simulink model "cesna_a_37"  (Simulink 7.6)
settings: Solver=ode45  StartTime=0.0  StopTime=200  RelTol=1e-3
model workspace (MAT data in the model file):
  CD_p : Simulink.Parameter (value not decoded)
  CL_p : Simulink.Parameter (value not decoded)
  CY_p : Simulink.Parameter (value not decoded)
  Clm_p : Simulink.Parameter (value not decoded)
  Cmm_p : Simulink.Parameter (value not decoded)
  Cnm_p : Simulink.Parameter (value not decoded)
  S : Simulink.Parameter (value not decoded)
  cbar : Simulink.Parameter (value not decoded)
  b : Simulink.Parameter (value not decoded)
  m : Simulink.Parameter (value not decoded)
  ho : Simulink.Parameter (value not decoded)
  Vo : Simulink.Parameter (value not decoded)
  Ts : Simulink.Parameter (value not decoded)
undefined symbols (not defined in the file): A, alpha_trim, B, C, D, F_T_trim
libraries: simulink x3, Airframes x1
(part 1 of 2)
settings Model: Creator=Administrator  LastModifiedBy=jporter
settings DebuggingCC: StrictBusMsg=Warning
settings SFSimCC: SimParseCustomCode=off

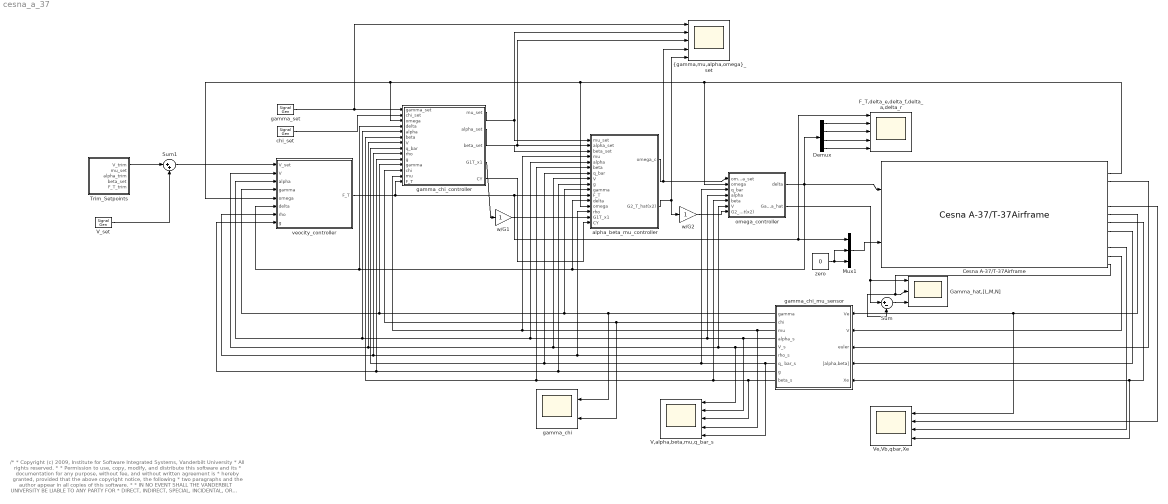
== system cesna_a_37 ==
  note: /*
      |  * Copyright (c) 2009, Institute for Software Integrated Systems, Vanderbilt University
      |  * All rights reserved.
      |  *
      |  * Permission to use, copy, modify, and distribute this software and its
      |  * documentation for any purpose, without fee, and without written agreement is
      |  * hereby granted, provided that the above copyright notice, the following
      |  * two paragraphs and the author appear in all copies of this software.
      |  *
      |  * IN NO EVENT SHALL THE VANDERBILT UNIVERSITY BE LIABLE TO ANY PARTY FOR
      |  * DIRECT, INDIRECT, SPECIAL, INCIDENTAL, OR CONSEQUENTIAL DAMAGES ARISING OUT
      |  * OF THE USE OF THIS SOFTWARE AND ITS DOCUMENTATION, EVEN IF THE VANDERBILT
      |  * UNIVERSITY HAS BEEN ADVISED OF THE POSSIBILITY OF SUCH DAMAGE.
      |  *
      |  * THE VANDERBILT UNIVERSITY SPECIFICALLY DISCLAIMS ANY WARRANTIES,
      |  * INCLUDING, BUT NOT LIMITED TO, THE IMPLIED WARRANTIES OF MERCHANTABILITY
      |  * AND FITNESS FOR A PARTICULAR PURPOSE.  THE SOFTWARE PROVIDED HEREUNDER IS
      |  * ON AN "AS IS" BASIS, AND THE VANDERBILT UNIVERSITY HAS NO OBLIGATION TO
      |  * PROVIDE MAINTENANCE, SUPPORT, UPDATES, ENHANCEMENTS, OR MODIFICATIONS.
      |  *
      |  * @author Nicholas Kottenstette
      |  * NB: Some of the atmospheric models (not including wind disturbance models) and drag-forc models including the
      | *  general aircraft interface description are for a large part a result of Giampiero Campa work with airlib, however,
      | *  equations of motion are determined using the standard 6-dof dynamic model after determening the respective
      | *  body forces applied to the aircraft not via the aerodynamic equations of motion involving angle of attack, slide-slip
      | * angle, etc.  Wind shear models and discrete-time gust models are based on the MIL–F–8785C specification.
      |  */
  Cesna A-37/T-37Airframe : Airframes/Cesna A-37//T-37Airframe  SystemSampleTime=-1  trim_enable=off  XYZe_0=[0,0,-1000]  V=Vo  Vb_0=Vo*[1,0,.0184]  euler_0=[0,.018,0]  omega_0=zeros(3,1)  M=.4535959237*6360  I=1.35581795*[7.99e3,0,2.34e2;0,3.33e3,0;2.34e2,0,1.12e4]  b=.3048*33.8  cbar=.3048*5.47  S=(.3048^2)*182  CG=[0,0,0]  CP=[0,0,0]  CD_p="[0.048,  0.384,  0,  0,  0]"  CL_p="[0.2,   5.15,    4.1,   0.5,   0]"  CY_p="[0,  -0.346,  -0.0827,  0.3,  0.0,  0.2]"  Clm_p="[0, -0.0944,  -0.442,  0.0926,  -0.181,  0.015]"  Cmm_p="[0.025, -0.7,  -14.9,  -1.12,  0]"  Cnm_p="[0,  0.1106, -0.0243,  -0.139,  0.0254,  -0.0365]"  delta_f=0  k_wind=on
  Demux : Demux
  F_T,delta_e,delta_f,delta_a,delta_r : Scope  NumInputPorts=5
      settings: YMin=0~-1.73472e-018~-1~-0.3~-0.175  YMax=17500~0.04~1~0.05~0.025  SaveName=actuator_s  SampleInput=on  SampleTime=0.05
  Gamma_hat,[L,M,N] : Scope  NumInputPorts=3
      settings: YMin=-1.5~-1.5~-3e-007  YMax=4~4~1.5e-007  SaveName=ScopeData12  SampleInput=on  SampleTime=0.01
  Mux1 : Mux  Inputs=3
  Sum : Sum  Inputs=|+-
  Sum1 : Sum  Inputs=|++
  Trim_Setpoints : Subsystem  mask{CD_p=CD_p, CL_p=CL_p, Cmm_p=Cmm_p, S=S, V=Vo, h=ho, m=m, delta_f=0}
      mask prompts: CD_p "Drag Parameters:CD_p=[CDo,CDa,CDq,CDde,CDin]"; CL_p "Lift Parameters:CL_p=[CLo,CLa,CLq,CLde,CLin]"; Cmm_p "m-moment (about-y_b) Parameters:Cmm_p=[Cmo,Cma,Cmq,Cmde,Cmin]"; S "Wing Area [S] (meters^2)"; V "Trim Velocity [V] (meters/s)"; h "Altitude [h] (meters)"; m "Mass [m] (kg)"; delta_f "delta_f [delta_f] (rad)"
      mask init:
      | [F_T_trim,alpha_trim,delta_e_trim,Sol] = fixed_wing_trim(CD_p,CL_p,Cmm_p,S,V,h,m,delta_f,[],false);
  V,alpha,beta,mu,q_bar_s : Scope  NumInputPorts=5
      settings: YMin=110~-0.05~-0.03~-0.5~6000  YMax=160~0.03~0.015~0.7~13000  SampleInput=on  SampleTime=0.04
  V_set : SignalGenerator  Amplitude=30  Frequency=.01
  Ve,Vb,qbar,Xe : Scope  NumInputPorts=4
      settings: YMin=-25~-25~12000~-1500  YMax=175~200~19000~4000  SaveName=ScopeData2  SampleInput=on  SampleTime=0.05
  alpha_beta_mu_controller : Subsystem  mask{CD_p=CD_p, CL_p=CL_p, CY_p=CY_p, S=S, b=b, cbar=cbar, m=m, K_2=[1,1,1]*1, Ts=Ts}
      mask prompts: CD_p "Drag Parameters:CD_p=[CDo,CDa,CDq,CDde,CDin]"; CL_p "Lift Parameters:CL_p=[CLo,CLa,CLq,CLde,CLin]"; CY_p "Y-Drag Parameters:CY_p=[CYo,CYb,CYp,CYr,CYda,CYdr]"; S "Wing Area [S] (meters^2)"; b "Wing Span [b] (meters)"; cbar "MAC [cbar] (meters)"; m "mass [m] (kg)"; Ts "Sample Time [Ts] (seconds)"
      mask init:
      | CDo=CD_p(1);
      | CDa=CD_p(2);
      | CDq=CD_p(3);
      | CDde=CD_p(4);
      | CDin=CD_p(5);
      | CLo=CL_p(1);
      | CLa=CL_p(2);
      | CLq=CL_p(3);
      | CLde=CL_p(4);
      | CLin=CL_p(5);
      | CYo=CY_p(1);
      | CYb=CY_p(2);
      | CYp=CY_p(3);
      | CYr=CY_p(4);
      | CYda=CY_p(5);
      | CYdr=CY_p(6);
  chi_set : SignalGenerator  Amplitude=.5  Frequency=.01
  gamma_chi : Scope  NumInputPorts=2
      settings: YMin=-0.1~-0.35  YMax=0.125~0.55  SaveName=ScopeData5  SampleInput=on  SampleTime=0.05
  gamma_chi_controller : Subsystem  mask{CL_p=CL_p, CY_p=CY_p, S=S, b=b, cbar=cbar, m=m, k_g=1, k_chi=.5, Ts=Ts}
      mask prompts: CL_p "Lift Parameters:CL_p=[CLo,CLa,CLq,CLde,CLin]"; CY_p "Y-Drag Parameters:CY_p=[CYo,CYb,CYp,CYr,CYda,CYdr]"; S "Wing Area [S] (meters^2)"; b "Wing Span [b] (meters)"; cbar "MAC [cbar] (meters)"; m "mass [m] (kg)"; Ts "Sample Period (s) [Ts]"
      mask init:
      | %CDo=CD_p(1);
      | %CDa=CD_p(2);
      | %CDq=CD_p(3);
      | %CDde=CD_p(4);
      | %CDin=CD_p(5);
      | CLo=CL_p(1);
      | CLa=CL_p(2);
      | CLq=CL_p(3);
      | CLde=CL_p(4);
      | CLin=CL_p(5);
      | CYo=CY_p(1);
      | CYb=CY_p(2);
      | CYp=CY_p(3);
      | CYr=CY_p(4);
      | CYda=CY_p(5);
      | CYdr=CY_p(6);
  gamma_chi_mu_sensor : Subsystem  mask{Ts=Ts}
      mask prompts: Ts "Sample Period (s) [Ts]"
  gamma_set : SignalGenerator  Amplitude=.1  Frequency=1/40
  omega_controller : Subsystem  mask{S=S, cbar=cbar, b=b, Clm_p=Clm_p, Cmm_p=Cmm_p, Cnm_p=Cnm_p, q_bar_nom=.5*1.225*Vo^2, k_o=[1,1,1]*1, Ts=Ts, I=1.35581795*[7.99e3,0,2.34e2;0,3.33e3,0;2.34e2,0,1.12e4]}
      mask prompts: S "Wing Area [S] (meters^2)"; cbar "MAC [cbar] (meters)"; b "Wing Span [b] (meters)"; Clm_p "l-moment (about x_b) Parameters: Clm_p=[Clo,Clb,Clp,Clr,Clda,Cldr]"; Cmm_p "m-moment (about-y_b) Parameters: Cmm_p=[Cmo,Cma,Cmq,Cmde,Cmin]"; Cnm_p "n-moment (about-z_b) Parameters:Cnm_p=[Cno,Cnb,Cnp,Cnr,Cnda,Cndr]"; Ts "Sample Period [Ts] (seconds)"; I "Inertial Matrix I"
      mask init:
      | Clo=Clm_p(1);
      | Clb=Clm_p(2);
      | Clp=Clm_p(3);
      | Clr=Clm_p(4);
      | Clda=Clm_p(5);
      | Cldr=Clm_p(6);
      | Cno=Cnm_p(1);
      | Cnb=Cnm_p(2);
      | Cnp=Cnm_p(3);
      | Cnr=Cnm_p(4);
      | Cnda=Cnm_p(5);
      | Cndr=Cnm_p(6);
      | Cmo=Cmm_p(1);
      | Cma=Cmm_p(2);
      | Cmq=Cmm_p(3);
      | Cmde=Cmm_p(4);
      | Cmin=Cmm_p(5);
  veocity_controller : Subsystem  mask{Ts=Ts, K_I=2, omega_d=1, CD_p=CD_p, CL_p=CL_p, Cmm_p=Cmm_p, S=S, V=Vo, h=ho, m=m, delta_f=0, cbar=cbar}
      mask prompts: Ts "Sample Period (s) [Ts]"; omega_d "omega_d (rad/s)"; CD_p "Drag Parameters:CD_p=[CDo,CDa,CDq,CDde,CDin]"; CL_p "Lift Parameters:CL_p=[CLo,CLa,CLq,CLde,CLin]"; Cmm_p "m-moment (about-y_b) Parameters:Cmm_p=[Cmo,Cma,Cmq,Cmde,Cmin]"; S "Wing Area (m^2): [S]"; V "Initial Trim Velocity [V] (meters/s)"; h "Initial Altitude [h] (meters)"; m "mass: (kg) [m]"; delta_f "delta_f [delta_f] (rad)"; cbar "MAC (m): [cbar]"
      mask init:
      | CDo=CD_p(1);
      | CDa=CD_p(2);
      | CDq=CD_p(3);
      | CDde=CD_p(4);
      | CDin=CD_p(5);
      | omega_n=pi/Ts;
      | [F_T_trim,alpha_trim,delta_e_trim,Sol] = fixed_wing_trim(CD_p,CL_p,Cmm_p,S,V,h,m,delta_f,[],false);
      | %Determine gravity and density at h
      | Po = 101325; %standard pressure [Pa]
      | To = 288.15; %standard temperature [Kelvin]
      | L = 6.5; %Kelvin/km
      | M = 28.9644; %gm/mol
      | R = 8.31432; %J/(mol-Kelvin)
      | g = 9.80665*((6356e3/(6356e3+h))^2);
      | T = To - 1.0e-3*L*h;
      | ps = Po*(T/To)^((g*M)/(R*L));   %Pressure at h
      | rho = ps/((1000*R/M)*T);
      | %Determine controller offset force
      | q_bar=.5*rho*V^2;
      | dF_T=-V*m*omega_d+q_bar*S*(CDa*alpha_trim+CDde*delta_e_trim+CDin*delta_f+CDo);
      | F_TI=F_T_trim-dF_T;
  w/G1 : Gain
  w/G2 : Gain
  zero : Constant  Value=0  SampleTime=Ts
  "{gamma,mu,alpha,omega}_set" : Scope  NumInputPorts=5
      settings: YMin=-0.1~-0.5~-0.03~-0.3~-0.3  YMax=0.1~0.9~0.03~0.3~0.3  SaveName=ScopeData4  SampleInput=on  SampleTime=0.05
  wires:
  gamma_chi_mu_sensor/1(gamma) -> veocity_controller/4(gamma), gamma_chi_controller/11(gamma), alpha_beta_mu_controller/10(gamma), gamma_chi/1
  Cesna A-37/T-37Airframe/7 -> gamma_chi_mu_sensor/1(Ve), Ve,Vb,qbar,Xe/1
  Cesna A-37/T-37Airframe/12 -> gamma_chi_mu_sensor/2(V)
  Cesna A-37/T-37Airframe/3 -> gamma_chi_mu_sensor/3(euler)
  Cesna A-37/T-37Airframe/9 -> gamma_chi_mu_sensor/4("[alpha,beta]")
  gamma_chi_mu_sensor/5(V_s) -> V,alpha,beta,mu,q_bar_s/1, alpha_beta_mu_controller/8(V), veocity_controller/2(V), gamma_chi_controller/7(V), omega_controller/6(V)
  gamma_chi_mu_sensor/4(alpha_s) -> omega_controller/4(alpha), alpha_beta_mu_controller/5(alpha), veocity_controller/3(alpha), gamma_chi_controller/5(alpha), V,alpha,beta,mu,q_bar_s/2
  Cesna A-37/T-37Airframe/8 -> gamma_chi_mu_sensor/5(Xe), Ve,Vb,qbar,Xe/4
  Cesna A-37/T-37Airframe/2 -> omega_controller/2(omega), alpha_beta_mu_controller/13(omega), veocity_controller/5(omega), gamma_chi_controller/3(omega)
  gamma_chi_mu_sensor/6(rho_s) -> alpha_beta_mu_controller/14(rho), veocity_controller/7(rho), gamma_chi_controller/9(rho)
  gamma_chi_mu_sensor/8(g) -> alpha_beta_mu_controller/9(g), veocity_controller/8(g), gamma_chi_controller/10(g)
  veocity_controller/1(F_T) -> alpha_beta_mu_controller/11(F_T), Mux1/1, F_T,delta_e,delta_f,delta_a,delta_r/1, gamma_chi_controller/14(F_T)
  omega_controller/1(delta) -> Cesna A-37/T-37Airframe/1, Demux/1, alpha_beta_mu_controller/12(delta), veocity_controller/6(delta), gamma_chi_controller/4(delta)
  gamma_chi_mu_sensor/7(q_ bar_s) -> V,alpha,beta,mu,q_bar_s/5, omega_controller/3(q_bar), alpha_beta_mu_controller/7(q_bar), gamma_chi_controller/8(q_bar)
  gamma_chi_mu_sensor/9(beta_s) -> omega_controller/5(beta), alpha_beta_mu_controller/6(beta), gamma_chi_controller/6(beta), V,alpha,beta,mu,q_bar_s/3
  alpha_beta_mu_controller/1(omega_c) -> omega_controller/1(omega_set), "{gamma,mu,alpha,omega}_set"/4
  gamma_chi_mu_sensor/3(mu) -> V,alpha,beta,mu,q_bar_s/4, alpha_beta_mu_controller/4(mu), gamma_chi_controller/13(mu)
  Demux/1 -> F_T,delta_e,delta_f,delta_a,delta_r/2
  Demux/2 -> F_T,delta_e,delta_f,delta_a,delta_r/3
  Demux/3 -> F_T,delta_e,delta_f,delta_a,delta_r/4
  Demux/4 -> F_T,delta_e,delta_f,delta_a,delta_r/5
  Cesna A-37/T-37Airframe/6 -> Ve,Vb,qbar,Xe/2
  Cesna A-37/T-37Airframe/11 -> Ve,Vb,qbar,Xe/3
  Mux1/1 -> Cesna A-37/T-37Airframe/2
  zero/1 -> Mux1/3, Mux1/2
  gamma_chi_mu_sensor/2(chi) -> gamma_chi/2, gamma_chi_controller/12(chi)
  gamma_chi_controller/2(alpha_set) -> alpha_beta_mu_controller/2(alpha_set), "{gamma,mu,alpha,omega}_set"/3
  gamma_chi_controller/1(mu_set) -> alpha_beta_mu_controller/1(mu_set), "{gamma,mu,alpha,omega}_set"/2
  gamma_chi_controller/3(beta_set) -> alpha_beta_mu_controller/3(beta_set)
  gamma_set/1 -> gamma_chi_controller/1(gamma_set), "{gamma,mu,alpha,omega}_set"/1
  chi_set/1 -> gamma_chi_controller/2(chi_set)
  Cesna A-37/T-37Airframe/13 -> Gamma_hat,[L,M,N]/2, Sum/2
  omega_controller/2(Gamma_hat) -> Gamma_hat,[L,M,N]/1, Sum/1
  Sum/1 -> Gamma_hat,[L,M,N]/3
  Trim_Setpoints/1(V_trim) -> Sum1/1
  Sum1/1 -> veocity_controller/1(V_set)
  V_set/1 -> Sum1/2
  gamma_chi_controller/4(G1T_x1) -> w/G1/1
  alpha_beta_mu_controller/2(G2_T_hat(x2)) -> "{gamma,mu,alpha,omega}_set"/5, w/G2/1
  w/G2/1 -> omega_controller/7(G2_T_hat(x2))
  w/G1/1 -> alpha_beta_mu_controller/15(G1T_x1)
  gamma_chi_controller/5(CY) -> alpha_beta_mu_controller/16(CY)

== system cesna_a_37/Trim_Setpoints ==
  Constant : Constant  Value=0
  V_trim_c : Constant  Value=V
  alpha_trim_c : Constant  Value=alpha_trim
  alpha_trim_c1 : Constant  Value=F_T_trim
  V_trim : Outport
  mu_set : Outport  Port=2
  alpha_trim : Outport  Port=3
  beta_set : Outport  Port=4
  F_T_trim : Outport  Port=5
  wires:
  Constant/1 -> mu_set/1, beta_set/1
  V_trim_c/1 -> V_trim/1
  alpha_trim_c/1 -> alpha_trim/1
  alpha_trim_c1/1 -> F_T_trim/1

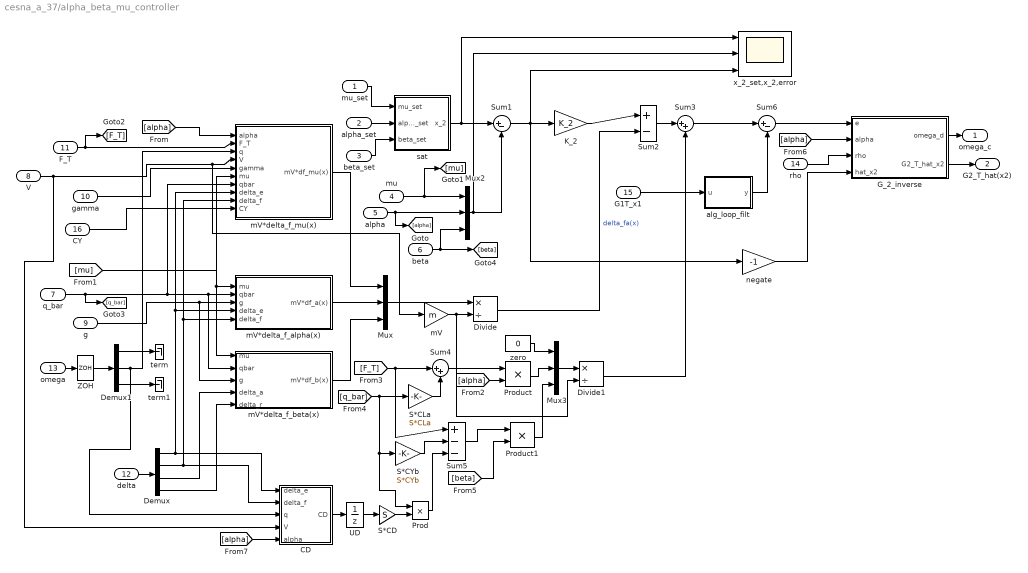
== system cesna_a_37/alpha_beta_mu_controller ==
  mu_set : Inport
  alpha_set : Inport  Port=2
  beta_set : Inport  Port=3
  mu : Inport  Port=4
  alpha : Inport  Port=5
  beta : Inport  Port=6
  q_bar : Inport  Port=7
  V : Inport  Port=8
  g : Inport  Port=9
  gamma : Inport  Port=10
  F_T : Inport  Port=11
  delta : Inport  Port=12
  omega : Inport  Port=13
  rho : Inport  Port=14
  G1T_x1 : Inport  Port=15
  CY : Inport  Port=16
  CD : Subsystem
  Demux : Demux
  Demux1 : Demux  Outputs=3
  Divide : Product  Inputs=*/
  Divide1 : Product  Inputs=*/
  G_2_inverse : Stateflow chart  TreatAsAtomicUnit=on
  K_2 : Gain  Gain=K_2
  Mux : Mux  Inputs=3
  Mux2 : Mux  Inputs=3
  Mux3 : Mux  Inputs=3
  Prod : Product  RndMeth=Zero
  Product : Product  RndMeth=Zero
  Product1 : Product  RndMeth=Zero
  S*CD : Gain  Gain=S
  S*CLa : Gain  Gain=S*CLa
  S*CYb : Gain  Gain=S*CYb
  Sum1 : Sum  Inputs=|+-
  Sum2 : Sum  Inputs=|+-
  Sum3 : Sum  Inputs=|++
  Sum4 : Sum  Inputs=|++
  Sum5 : Sum  Inputs=|+--
  Sum6 : Sum  Inputs=|+-
  UD : UnitDelay  SampleTime=-1
  ZOH : ZeroOrderHold  SampleTime=Ts
  alg_loop_filt : Subsystem
  mV : Gain  Gain=m
  mV*delta_f_alpha(x) : Subsystem
  mV*delta_f_beta(x) : Subsystem
  mV*delta_f_mu(x) : Subsystem
  negate : Gain  Gain=-1
  sat : Subsystem
  term : Terminator
  term1 : Terminator
  x_2_set,x_2,error : Scope  NumInputPorts=3
      settings: YMin=-0.4~-0.4~-0.15  YMax=0.6~0.5~0.45  SaveName=x2_s  SampleInput=on  SampleTime=0.05
  zero : Constant  Value=0
  omega_c : Outport
  G2_T_hat(x2) : Outport  Port=2
  wires:
  g/1 -> mV*delta_f_alpha(x)/3(g), mV*delta_f_beta(x)/3(g)
  q_bar/1 -> mV*delta_f_alpha(x)/2(qbar), mV*delta_f_beta(x)/2(qbar), mV*delta_f_mu(x)/7(qbar), [q_bar]
  delta/1 -> Demux/1
  Demux/1 -> mV*delta_f_alpha(x)/4(delta_e), mV*delta_f_mu(x)/8(delta_e), CD/1(delta_e)
  Demux/2 -> mV*delta_f_alpha(x)/5(delta_f), mV*delta_f_mu(x)/9(delta_f), CD/2(delta_f)
  Demux/3 -> mV*delta_f_beta(x)/4(delta_a)
  Demux/4 -> mV*delta_f_beta(x)/5(delta_r)
  V/1 -> mV*delta_f_mu(x)/4(V), mV/1, CD/4(V)
  F_T/1 -> mV*delta_f_mu(x)/2(F_T), [F_T]
  gamma/1 -> mV*delta_f_mu(x)/5(gamma)
  omega/1 -> ZOH/1
  Demux1/2 -> mV*delta_f_mu(x)/3(q), CD/3(q)
  mV*delta_f_alpha(x)/1(mV*df_a(x)) -> Mux/2
  mV*delta_f_mu(x)/1(mV*df_mu(x)) -> Mux/1
  mV*delta_f_beta(x)/1(mV*df_b(x)) -> Mux/3
  Mux/1 -> Divide/1
  mV/1 -> Divide/2, Divide1/2
  alpha/1 -> [alpha], Mux2/2
  beta/1 -> [beta], Mux2/3
  mu/1 -> [mu], Mux2/1
  Mux2/1 -> x_2_set,x_2,error/2, Sum1/2
  Sum1/1 -> K_2/1, negate/1, x_2_set,x_2,error/3
  G_2_inverse/1(omega_d) -> omega_c/1
  rho/1 -> G_2_inverse/3(rho)
  ZOH/1 -> Demux1/1
  Demux1/3 -> term1/1
  Demux1/1 -> term/1
  [alpha] -> mV*delta_f_mu(x)/1(alpha)
  [mu] -> mV*delta_f_mu(x)/6(mu), mV*delta_f_beta(x)/1(mu), mV*delta_f_alpha(x)/1(mu)
  Sum2/1 -> Sum3/1
  zero/1 -> Mux3/1
  Mux3/1 -> Divide1/1
  Divide1/1 -> Sum3/2
  [q_bar] -> S*CLa/1, S*CYb/1, Prod/1
  [F_T] -> Sum5/1, Sum4/1
  S*CLa/1 -> Sum4/2
  Sum4/1 -> Product/1
  Product/1 -> Mux3/2
  [alpha] -> Product/2
  S*CYb/1 -> Sum5/2
  [beta] -> Product1/2
  Product1/1 -> Mux3/3
  Sum5/1 -> Product1/1
  [alpha] -> G_2_inverse/2(alpha)
  mu_set/1 -> sat/1(mu_set)
  alpha_set/1 -> sat/2(alpha_set)
  beta_set/1 -> sat/3(beta_set)
  Sum3/1 -> Sum6/1
  Sum6/1 -> G_2_inverse/1(e)
  G_2_inverse/2(G2_T_hat_x2) -> G2_T_hat(x2)/1
  negate/1 -> G_2_inverse/4(hat_x2)
  CY/1 -> mV*delta_f_mu(x)/10(CY)
  alg_loop_filt/1(y) -> Sum6/2
  G1T_x1/1 -> alg_loop_filt/1(u)
  CD/1(CD) -> UD/1
  [alpha] -> CD/5(alpha)
  K_2/1 -> Sum2/1
  Divide/1 -> Sum2/2  "delta_fa(x)"
  sat/1(x_2) -> Sum1/1, x_2_set,x_2,error/1
  S*CD/1 -> Prod/2
  Prod/1 -> Sum5/3
  UD/1 -> S*CD/1

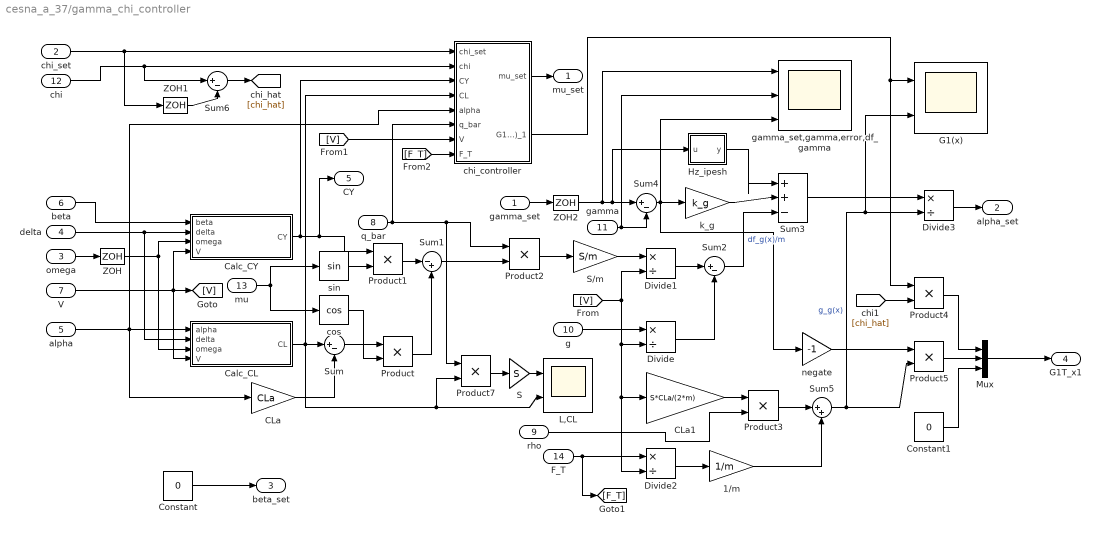
== system cesna_a_37/gamma_chi_controller ==
  gamma_set : Inport
  chi_set : Inport  Port=2
  omega : Inport  Port=3
  delta : Inport  Port=4
  alpha : Inport  Port=5
  beta : Inport  Port=6
  V : Inport  Port=7
  q_bar : Inport  Port=8
  rho : Inport  Port=9
  g : Inport  Port=10
  gamma : Inport  Port=11
  chi : Inport  Port=12
  mu : Inport  Port=13
  F_T : Inport  Port=14
  1/m : Gain  Gain=1/m
  CLa : Gain  Gain=CLa
  CLa1 : Gain  Gain=S*CLa/(2*m)
  Calc_CL : Subsystem
  Calc_CY : Subsystem
  Constant : Constant  Value=0
  Constant1 : Constant  Value=0
  Divide{,1..3} (4 alike) : Product  Inputs=*/
  G1(x) : Scope  NumInputPorts=2
      settings: YMin=0.055~1.65  YMax=0.13~2.4  SaveName=ScopeData10  SampleInput=on  SampleTime=0.05
  Hz_ipesh : Subsystem  mask{num=[1,0], den=[10*Ts/pi,1], Ts=Ts, y0=0}
      mask prompts: num "Hs num [num]"; den "Hs den [den]"; Ts "Sample Period (s) [Ts]"; y0 "y0 (N)"
      mask init:
      | Hs=tf(num,den);
      | Hz=ipesh_transform(Hs,Ts);
      | [A,B,C,D]=tf2ss(Hz.num{1},Hz.den{1});
      | x0=y0/C;
  L,CL : Scope  NumInputPorts=2
      settings: YMin=-5000~-0.025  YMax=70000~0.35  SaveName=ScopeData14  SampleInput=on  SampleTime=0.05
  Mux : Mux  Inputs=3
  Product{,1..5,7} (7 alike) : Product  RndMeth=Zero
  S : Gain  Gain=S
  S/m : Gain  Gain=S/m
  Sum{,2,4,6} (4 alike) : Sum  Inputs=|+-
  Sum1 : Sum  Inputs=|-+
  Sum3 : Sum  Inputs=|++-
  Sum5 : Sum  Inputs=|++
  ZOH : ZeroOrderHold  SampleTime=Ts
  ZOH1 : ZeroOrderHold  SampleTime=Ts
  ZOH2 : ZeroOrderHold  SampleTime=Ts
  chi_controller : Subsystem
  cos : Trigonometry  Operator=cos
  gamma_set,gamma,error,df_gamma : Scope  NumInputPorts=3
      settings: YMin=-0.1~-0.125~-0.015  YMax=0.1~0.125~0.04  SaveName=gamma_s  SampleInput=on  SampleTime=0.05
  k_g : Gain  Gain=k_g
  negate : Gain  Gain=-1
  sin : Trigonometry
  mu_set : Outport
  alpha_set : Outport  Port=2
  beta_set : Outport  Port=3
  G1T_x1 : Outport  Port=4
  CY : Outport  Port=5
  wires:
  alpha/1 -> Calc_CL/1(alpha), CLa/1, chi_controller/5(alpha)
  delta/1 -> Calc_CY/2(delta), Calc_CL/2(delta)
  beta/1 -> Calc_CY/1(beta)
  omega/1 -> ZOH/1
  V/1 -> Calc_CL/4(V), Calc_CY/4(V), [V]
  Calc_CL/1(CL) -> chi_controller/4(CL), Sum/1, L,CL/2, Product7/2
  CLa/1 -> Sum/2
  g/1 -> Divide/1
  Sum/1 -> Product/1
  mu/1 -> sin/1, cos/1
  cos/1 -> Product/2
  sin/1 -> Product1/2
  Calc_CY/1(CY) -> chi_controller/3(CY), Product1/1, CY/1
  Product1/1 -> Sum1/1
  Product/1 -> Sum1/2
  Sum1/1 -> Product2/2
  q_bar/1 -> chi_controller/6(q_bar), Product2/1, Product7/1
  Product2/1 -> S/m/1
  S/m/1 -> Divide1/1
  [V] -> Divide1/2, Divide/2, CLa1/1, Divide2/2
  Divide1/1 -> Sum2/1
  Divide/1 -> Sum2/2
  gamma_set/1 -> ZOH2/1
  gamma/1 -> gamma_set,gamma,error,df_gamma/2, Sum4/2
  Sum4/1 -> k_g/1, gamma_set,gamma,error,df_gamma/3, negate/1
  F_T/1 -> Divide2/1, [F_T]
  Divide2/1 -> 1/m/1
  1/m/1 -> Sum5/2
  CLa1/1 -> Product3/1
  rho/1 -> Product3/2
  Product3/1 -> Sum5/1
  Sum3/1 -> Divide3/1
  Sum5/1 -> Divide3/2, G1(x)/2, Product5/2  "g_g(x)"
  Divide3/1 -> alpha_set/1
  chi_set/1 -> chi_controller/1(chi_set), ZOH1/1
  chi/1 -> chi_controller/2(chi), Sum6/1
  Constant/1 -> beta_set/1
  ZOH/1 -> Calc_CY/3(omega), Calc_CL/3(omega)
  ZOH2/1 -> gamma_set,gamma,error,df_gamma/1, Sum4/1, Hz_ipesh/1(u)
  [V] -> chi_controller/7(V)
  [F_T] -> chi_controller/8(F_T)
  chi_controller/1(mu_set) -> mu_set/1
  Sum2/1 -> Sum3/3  "df_g(x)/m"
  k_g/1 -> Sum3/2
  Hz_ipesh/1(y) -> Sum3/1
  chi_controller/2(G1(x)_1) -> G1(x)/1, Product4/1
  [chi_hat] -> Product4/2
  negate/1 -> Product5/1
  Mux/1 -> G1T_x1/1
  Product4/1 -> Mux/1
  Product5/1 -> Mux/2
  Constant1/1 -> Mux/3
  Sum6/1 -> [chi_hat]
  ZOH1/1 -> Sum6/2
  Product7/1 -> S/1
  S/1 -> L,CL/1

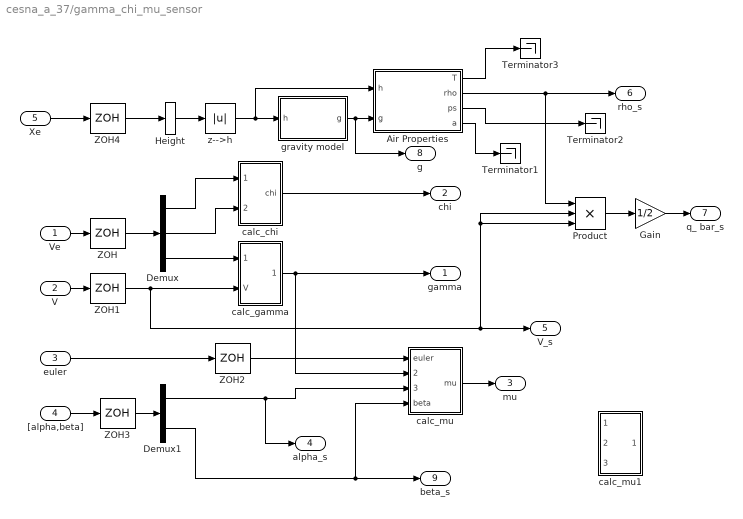
== system cesna_a_37/gamma_chi_mu_sensor ==
  Ve : Inport
  V : Inport  Port=2
  euler : Inport  Port=3
  "[alpha,beta]" : Inport  Port=4
  Xe : Inport  Port=5
  Air Properties : Stateflow chart  TreatAsAtomicUnit=on
  Demux : Demux  Outputs=3
  Demux1 : Demux  Outputs=2
  Gain : Gain  Gain=1/2
  Height : Selector  InputPortWidth=3  IndexOptions=Index vector (dialog)  Indices=[3]  OutputSizes=1
  Product : Product  Inputs=3  RndMeth=Zero
  Terminator1 : Terminator
  Terminator2 : Terminator
  Terminator3 : Terminator
  ZOH{,1..4} (5 alike) : ZeroOrderHold  SampleTime=Ts
  calc_chi : Subsystem
  calc_gamma : Subsystem
  calc_mu : Subsystem
  calc_mu1 : Subsystem
  gravity model : Subsystem
  z-->h : Abs  SaturateOnIntegerOverflow=on
  gamma : Outport
  chi : Outport  Port=2
  mu : Outport  Port=3
  alpha_s : Outport  Port=4
  V_s : Outport  Port=5
  rho_s : Outport  Port=6
  q_ bar_s : Outport  Port=7
  g : Outport  Port=8
  beta_s : Outport  Port=9
  wires:
  Ve/1 -> ZOH/1
  Demux/3 -> calc_gamma/1(v_I3)
  V/1 -> ZOH1/1
  calc_gamma/1(gamma) -> gamma/1, calc_mu/2(gamma)
  Demux/1 -> calc_chi/1(v_I1)
  Demux/2 -> calc_chi/2(v_I2)
  calc_chi/1(chi) -> chi/1
  euler/1 -> ZOH2/1
  calc_mu/1(mu) -> mu/1
  ZOH/1 -> Demux/1
  ZOH1/1 -> calc_gamma/2(V), V_s/1, Product/2, Product/3
  ZOH2/1 -> calc_mu/1(euler)
  "[alpha,beta]"/1 -> ZOH3/1
  Demux1/1 -> calc_mu/3(alpha), alpha_s/1
  Height/1 -> z-->h/1
  Xe/1 -> ZOH4/1
  ZOH4/1 -> Height/1
  z-->h/1 -> Air Properties/1(h), gravity model/1(h)
  gravity model/1(g) -> Air Properties/2(g), g/1
  Air Properties/2(rho) -> rho_s/1, Product/1
  Air Properties/4(a) -> Terminator1/1
  Air Properties/3(ps) -> Terminator2/1
  Air Properties/1(T) -> Terminator3/1
  Product/1 -> Gain/1
  Gain/1 -> q_ bar_s/1
  ZOH3/1 -> Demux1/1
  Demux1/2 -> beta_s/1, calc_mu/4(beta)

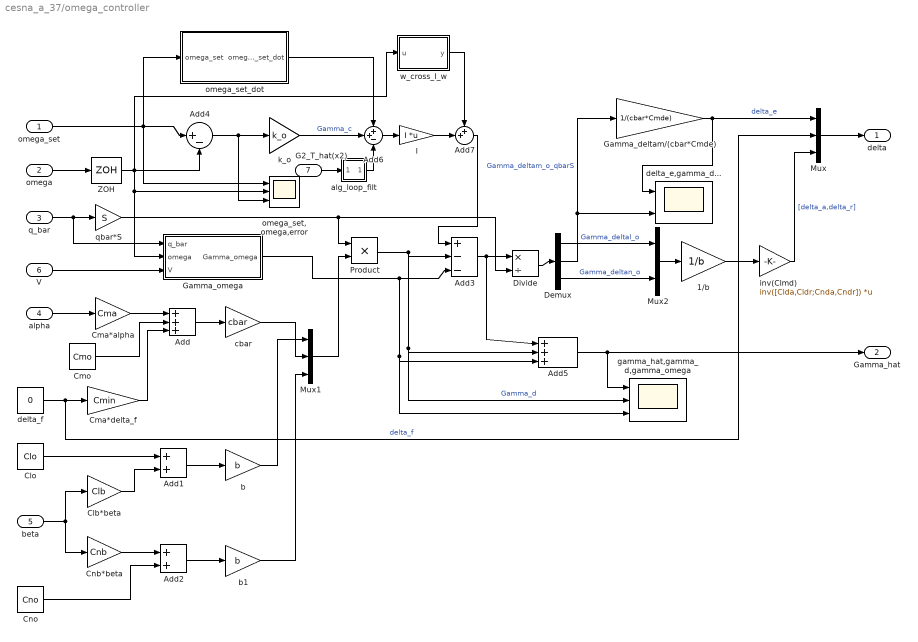
== system cesna_a_37/omega_controller ==
  omega_set : Inport
  omega : Inport  Port=2
  q_bar : Inport  Port=3
  alpha : Inport  Port=4
  beta : Inport  Port=5
  V : Inport  Port=6
  G2_T_hat(x2) : Inport  Port=7
  1/b : Gain  Gain=1/b
  Add : Sum  Inputs=+++
  Add1 : Sum
  Add2 : Sum
  Add3 : Sum  Inputs=+--|
  Add4 : Sum  Inputs=|+-
  Add5 : Sum  Inputs=+++|
  Add6 : Sum  Inputs=++-
  Add7 : Sum  Inputs=++|
  Clb*beta : Gain  Gain=Clb
  Clo : Constant  Value=Clo  SampleTime=Ts
  Cma*alpha : Gain  Gain=Cma
  Cma*delta_f : Gain  Gain=Cmin
  Cmo : Constant  Value=Cmo  SampleTime=Ts
  Cnb*beta : Gain  Gain=Cnb
  Cno : Constant  Value=Cno  SampleTime=Ts
  Demux : Demux  Outputs=3
  Divide : Product  Inputs=*/
  Gamma_deltam/(cbar*Cmde) : Gain  Gain=1/(cbar*Cmde)
  Gamma_omega : Stateflow chart  TreatAsAtomicUnit=on
  I : Gain  Gain=I  Multiplication=Matrix(K*u)
  Mux : Mux  Inputs=[1,1,2]
  Mux1 : Mux  Inputs=3
  Mux2 : Mux  Inputs=2
  Product : Product  RndMeth=Zero
  ZOH : ZeroOrderHold  SampleTime=Ts
  alg_loop_filt : Subsystem
  b : Gain  Gain=b
  b1 : Gain  Gain=b
  cbar : Gain  Gain=cbar
  delta_e,gamma_d... : Scope  NumInputPorts=2
      settings: YMin=-5~-5  YMax=5~5  SaveName=ScopeData3  SampleInput=on  SampleTime=0.01
  delta_f : Constant  Value=0  SampleTime=Ts
  gamma_hat,gamma_d,gamma_omega : Scope  NumInputPorts=3
      settings: YMin=-5~-5~-5  YMax=5~5~5  SaveName=ScopeData13  SampleInput=on  SampleTime=0.01
  inv(Clmd) : Gain  Gain=inv([Clda,Cldr;Cnda,Cndr])  Multiplication=Matrix(K*u)
  k_o : Gain  Gain=k_o
  "omega_set, omega,error" : Scope  NumInputPorts=3
      settings: YMin=-0.15~-0.15~-0.2  YMax=0.45~0.5~0.15  SaveName=omega_s  SampleInput=on  SampleTime=0.05
  omega_set_dot : Subsystem
  qbar*S : Gain  Gain=S
  w_cross_I_w : Stateflow chart  TreatAsAtomicUnit=on
  delta : Outport
  Gamma_hat : Outport  Port=2
  wires:
  omega/1 -> ZOH/1
  omega_set/1 -> Add4/1, "omega_set, omega,error"/1, omega_set_dot/1(omega_set)
  q_bar/1 -> qbar*S/1, Gamma_omega/1(q_bar)
  alpha/1 -> Cma*alpha/1
  Cma*alpha/1 -> Add/1
  Cmo/1 -> Add/2
  delta_f/1 -> Cma*delta_f/1, Mux/2  "delta_f"
  Cma*delta_f/1 -> Add/3
  Add/1 -> cbar/1
  cbar/1 -> Mux1/2
  Mux1/1 -> Product/2
  qbar*S/1 -> Product/1, Divide/2
  Clo/1 -> Add1/1
  beta/1 -> Clb*beta/1, Cnb*beta/1
  Clb*beta/1 -> Add1/2
  Cnb*beta/1 -> Add2/1
  Cno/1 -> Add2/2
  Add1/1 -> b/1
  Add2/1 -> b1/1
  b/1 -> Mux1/1
  b1/1 -> Mux1/3
  Product/1 -> Add3/2, Add5/2, gamma_hat,gamma_d,gamma_omega/2  "Gamma_d"
  ZOH/1 -> Add4/2, "omega_set, omega,error"/2, Gamma_omega/2(omega), w_cross_I_w/1(u)
  Add4/1 -> "omega_set, omega,error"/3, k_o/1
  Mux/1 -> delta/1
  Divide/1 -> Demux/1
  Gamma_deltam/(cbar*Cmde)/1 -> Mux/1, delta_e,gamma_d.../1  "delta_e"
  Demux/2 -> Gamma_deltam/(cbar*Cmde)/1, delta_e,gamma_d.../2  "Gamma_deltam_o_qbarS"
  Demux/1 -> Mux2/1  "Gamma_deltal_o"
  Demux/3 -> Mux2/2  "Gamma_deltan_o"
  Mux2/1 -> 1/b/1
  1/b/1 -> inv(Clmd)/1
  inv(Clmd)/1 -> Mux/3  "[delta_a,delta_r]"
  V/1 -> Gamma_omega/3(V)
  Gamma_omega/1(Gamma_omega) -> Add3/3, Add5/3, gamma_hat,gamma_d,gamma_omega/3
  Add5/1 -> Gamma_hat/1, gamma_hat,gamma_d,gamma_omega/1
  k_o/1 -> Add6/2  "Gamma_c"
  Add6/1 -> I/1
  omega_set_dot/1(omega_set_dot) -> Add6/1
  G2_T_hat(x2)/1 -> alg_loop_filt/1(u)
  alg_loop_filt/1(y) -> Add6/3
  Add3/1 -> Divide/1, Add5/1
  I/1 -> Add7/2
  Add7/1 -> Add3/1
  w_cross_I_w/1(y) -> Add7/1

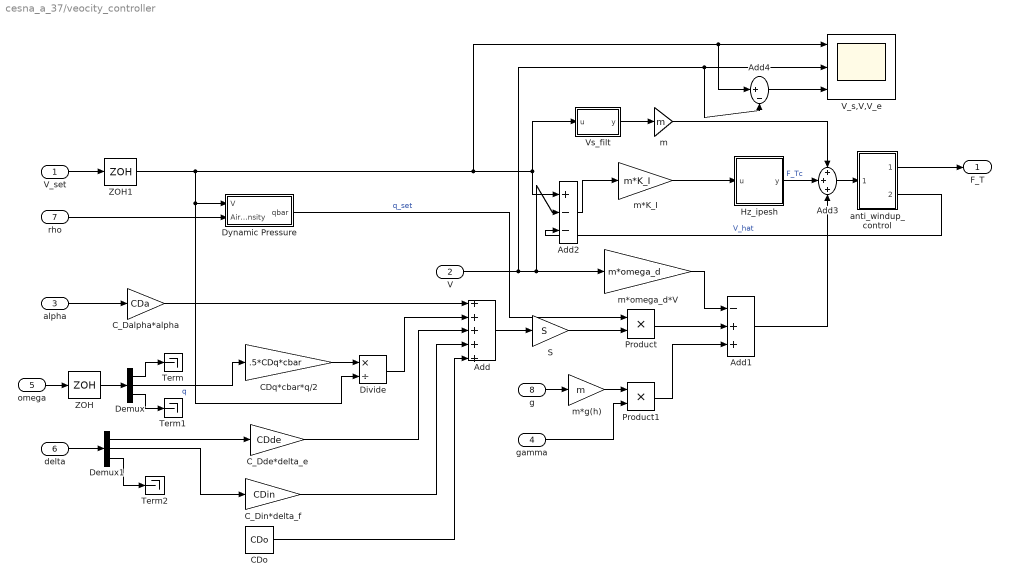
== system cesna_a_37/veocity_controller ==
  V_set : Inport
  V : Inport  Port=2
  alpha : Inport  Port=3
  gamma : Inport  Port=4
  omega : Inport  Port=5
  delta : Inport  Port=6
  rho : Inport  Port=7
  g : Inport  Port=8
  Add : Sum  Inputs=+++++
  Add1 : Sum  Inputs=-++
  Add2 : Sum  Inputs=|+--
  Add3 : Sum  Inputs=+++
  Add4 : Sum  Inputs=|+-
  CDo : Constant  Value=CDo  SampleTime=Ts
  CDq*cbar*q/2 : Gain  Gain=.5*CDq*cbar
  C_Dalpha*alpha : Gain  Gain=CDa
  C_Dde*delta_e : Gain  Gain=CDde
  C_Din*delta_f : Gain  Gain=CDin
  Demux : Demux  Outputs=3
  Demux1 : Demux  Outputs=[1,1,2]
  Divide : Product  Inputs=*/
  Dynamic Pressure : Subsystem  mask(Dynamic Pressure){}
      mask help: Compute dynamic pressure using velocity and air density.
      mask init:
      | aeroicon('aeroblk');
      mask Help: eval('asbhelp');
      mask Display:
      | port_label('input',1,'V','texmode','on');
      | port_label('input',2,'\rho','texmode','on');
      | port_label('output',1,'q','texmode','on');
      | disp('^1/_2 \rhoV^2','texmode','on');
  Hz_ipesh : Subsystem  mask{num=[1,omega_d], den=[1,0], Ts=Ts, y0=0}
      mask prompts: num "Hs num [num]"; den "Hs den [den]"; Ts "Sample Period (s) [Ts]"; y0 "y0 (N)"
      mask init:
      | Hs=tf(num,den);
      | Hz=ipesh_transform(Hs,Ts);
      | [A,B,C,D]=tf2ss(Hz.num{1},Hz.den{1});
      | x0=y0/C;
  Product : Product  RndMeth=Zero
  Product1 : Product  RndMeth=Zero
  S : Gain  Gain=S
  Term : Terminator
  Term1 : Terminator
  Term2 : Terminator
  V_s,V,V_e : Scope  NumInputPorts=3
      settings: TimeRange=200  YMin=130~135~-13  YMax=160~162.5~0  SaveName=V_s  SampleInput=on  SampleTime=0.05
  Vs_filt : Subsystem  mask{num=[1], den=[Ts/(10*pi),1], Ts=Ts, u0=Vo, y0=Vo}
      mask prompts: num "Hs num [num]"; den "Hs den [den]"; Ts "Sample Period (s) [Ts]"; u0 "u0 (m/s)"; y0 "yo (m/s^2)"
      mask init:
      | Hs=tf(num,den);
      | Hz=ipesh_transform(Hs,Ts);
      | [A,B,C,D]=tf2ss(Hz.num{1},Hz.den{1});
      | x0=(y0-D*u0)/C;
  ZOH : ZeroOrderHold  SampleTime=Ts
  ZOH1 : ZeroOrderHold  SampleTime=Ts
  anti_windup_control : Subsystem
  m : Gain  Gain=m
  m*K_I : Gain  Gain=m*K_I
  m*g(h) : Gain  Gain=m
  m*omega_d*V : Gain  Gain=m*omega_d
  F_T : Outport
  wires:
  omega/1 -> ZOH/1
  V_set/1 -> ZOH1/1
  rho/1 -> Dynamic Pressure/2(Air Density)
  ZOH1/1 -> Dynamic Pressure/1(V), Divide/2, Add2/1, Vs_filt/1(u), V_s,V,V_e/1, Add4/1
  alpha/1 -> C_Dalpha*alpha/1
  ZOH/1 -> Demux/1
  Demux/2 -> CDq*cbar*q/2/1  "q"
  CDq*cbar*q/2/1 -> Divide/1
  delta/1 -> Demux1/1
  Demux1/1 -> C_Dde*delta_e/1
  Demux1/2 -> C_Din*delta_f/1
  C_Dalpha*alpha/1 -> Add/1
  Divide/1 -> Add/2
  C_Dde*delta_e/1 -> Add/3
  C_Din*delta_f/1 -> Add/4
  CDo/1 -> Add/5
  Add/1 -> S/1
  S/1 -> Product/2
  Dynamic Pressure/1(qbar) -> Product/1  "q_set"
  g/1 -> m*g(h)/1
  m*g(h)/1 -> Product1/1
  gamma/1 -> Product1/2
  Product/1 -> Add1/2
  Product1/1 -> Add1/3
  V/1 -> m*omega_d*V/1, Add2/2, V_s,V,V_e/2, Add4/2
  m*omega_d*V/1 -> Add1/1
  Add2/1 -> m*K_I/1
  Demux1/3 -> Term2/1
  Demux/1 -> Term/1
  Demux/3 -> Term1/1
  m*K_I/1 -> Hz_ipesh/1(u)
  Vs_filt/1(y) -> m/1
  anti_windup_control/2(Out2) -> Add2/3  "V_hat"
  Add3/1 -> anti_windup_control/1(In1)
  anti_windup_control/1(Out1) -> F_T/1
  Add4/1 -> V_s,V,V_e/3
  Hz_ipesh/1(y) -> Add3/2  "F_Tc"
  Add1/1 -> Add3/3
  m/1 -> Add3/1

== system cesna_a_37/alpha_beta_mu_controller/CD ==
  delta_e : Inport
  delta_f : Inport  Port=2
  q : Inport  Port=3
  V : Inport  Port=4
  alpha : Inport  Port=5
  Add : Sum  Inputs=+++++
  CDa*alpha : Gain  Gain=CDa
  CDde*delta_e : Gain  Gain=CDde
  CDin*delta_f : Gain  Gain=CDin
  CDo : Constant  Value=CDo
  Divide : Product  Inputs=*/
  q*cbar*CDq/2 : Gain  Gain=cbar*CDq/2
  CD : Outport
  wires:
  CDo/1 -> Add/1
  CDde*delta_e/1 -> Add/2
  delta_e/1 -> CDde*delta_e/1
  alpha/1 -> CDa*alpha/1
  Add/1 -> CD/1
  delta_f/1 -> CDin*delta_f/1
  CDin*delta_f/1 -> Add/3
  CDa*alpha/1 -> Add/4
  q/1 -> q*cbar*CDq/2/1
  q*cbar*CDq/2/1 -> Divide/1
  V/1 -> Divide/2
  Divide/1 -> Add/5

== system cesna_a_37/alpha_beta_mu_controller/alg_loop_filt ==
  u : Inport
  Demux : Demux  Outputs=3
  Hz_ipesh : Subsystem  mask{num=[1], den=[10*Ts/pi,1], Ts=Ts, y0=0}
      mask prompts: num "Hs num [num]"; den "Hs den [den]"; Ts "Sample Period (s) [Ts]"; y0 "y0 (N)"
      mask init:
      | Hs=tf(num,den);
      | Hz=ipesh_transform(Hs,Ts);
      | [A,B,C,D]=tf2ss(Hz.num{1},Hz.den{1});
      | x0=y0/C;
  Hz_ipesh1 : Subsystem  mask{num=[1,0], den=[10*Ts/pi,1], Ts=Ts, y0=0}
      mask prompts: num "Hs num [num]"; den "Hs den [den]"; Ts "Sample Period (s) [Ts]"; y0 "y0 (N)"
      mask init:
      | Hs=tf(num,den);
      | Hz=ipesh_transform(Hs,Ts);
      | [A,B,C,D]=tf2ss(Hz.num{1},Hz.den{1});
      | x0=y0/C;
  Hz_ipesh2 : Subsystem  mask{num=[1,0], den=[10*Ts/pi,1], Ts=Ts, y0=0}
      mask prompts: num "Hs num [num]"; den "Hs den [den]"; Ts "Sample Period (s) [Ts]"; y0 "y0 (N)"
      mask init:
      | Hs=tf(num,den);
      | Hz=ipesh_transform(Hs,Ts);
      | [A,B,C,D]=tf2ss(Hz.num{1},Hz.den{1});
      | x0=y0/C;
  Mux2 : Mux  Inputs=3
  Unit Delay : UnitDelay  SampleTime=-1
  y : Outport
  wires:
  Mux2/1 -> y/1
  Hz_ipesh2/1(y) -> Mux2/3
  Demux/3 -> Hz_ipesh2/1(u)
  Hz_ipesh1/1(y) -> Mux2/2
  Demux/2 -> Hz_ipesh1/1(u)
  Hz_ipesh/1(y) -> Mux2/1
  Demux/1 -> Hz_ipesh/1(u)
  u/1 -> Unit Delay/1
  Unit Delay/1 -> Demux/1

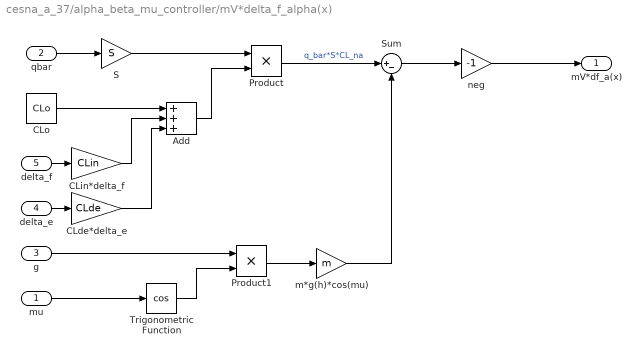
== system cesna_a_37/alpha_beta_mu_controller/mV*delta_f_alpha(x) ==
  mu : Inport
  qbar : Inport  Port=2
  g : Inport  Port=3
  delta_e : Inport  Port=4
  delta_f : Inport  Port=5
  Add : Sum  Inputs=+++
  CLde*delta_e : Gain  Gain=CLde
  CLin*delta_f : Gain  Gain=CLin
  CLo : Constant  Value=CLo
  Product : Product  RndMeth=Zero
  Product1 : Product  RndMeth=Zero
  S : Gain  Gain=S
  Sum : Sum  Inputs=|+-
  Trigonometric Function : Trigonometry  Operator=cos
  m*g(h)*cos(mu) : Gain  Gain=m
  neg : Gain  Gain=-1
  mV*df_a(x) : Outport
  wires:
  qbar/1 -> S/1
  S/1 -> Product/1
  Add/1 -> Product/2
  CLo/1 -> Add/1
  CLin*delta_f/1 -> Add/2
  delta_f/1 -> CLin*delta_f/1
  delta_e/1 -> CLde*delta_e/1
  CLde*delta_e/1 -> Add/3
  Product/1 -> Sum/1  "q_bar*S*CL_na"
  g/1 -> Product1/1
  mu/1 -> Trigonometric Function/1
  Trigonometric Function/1 -> Product1/2
  Product1/1 -> m*g(h)*cos(mu)/1
  m*g(h)*cos(mu)/1 -> Sum/2
  Sum/1 -> neg/1
  neg/1 -> mV*df_a(x)/1

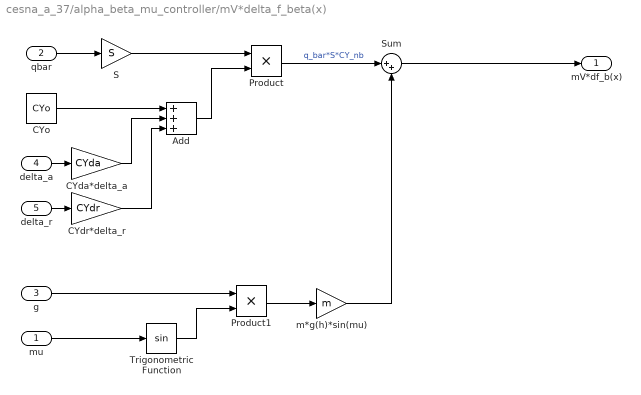
== system cesna_a_37/alpha_beta_mu_controller/mV*delta_f_beta(x) ==
  mu : Inport
  qbar : Inport  Port=2
  g : Inport  Port=3
  delta_a : Inport  Port=4
  delta_r : Inport  Port=5
  Add : Sum  Inputs=+++
  CYda*delta_a : Gain  Gain=CYda
  CYdr*delta_r : Gain  Gain=CYdr
  CYo : Constant  Value=CYo
  Product : Product  RndMeth=Zero
  Product1 : Product  RndMeth=Zero
  S : Gain  Gain=S
  Sum : Sum  Inputs=|++
  Trigonometric Function : Trigonometry
  m*g(h)*sin(mu) : Gain  Gain=m
  mV*df_b(x) : Outport
  wires:
  Sum/1 -> mV*df_b(x)/1
  m*g(h)*sin(mu)/1 -> Sum/2
  Product1/1 -> m*g(h)*sin(mu)/1
  Trigonometric Function/1 -> Product1/2
  mu/1 -> Trigonometric Function/1
  g/1 -> Product1/1
  Product/1 -> Sum/1  "q_bar*S*CY_nb"
  CYdr*delta_r/1 -> Add/3
  delta_r/1 -> CYdr*delta_r/1
  delta_a/1 -> CYda*delta_a/1
  CYda*delta_a/1 -> Add/2
  CYo/1 -> Add/1
  Add/1 -> Product/2
  S/1 -> Product/1
  qbar/1 -> S/1

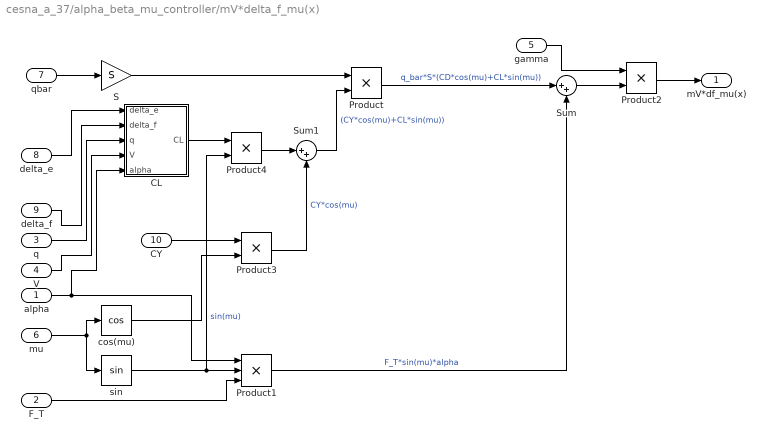
== system cesna_a_37/alpha_beta_mu_controller/mV*delta_f_mu(x) ==
  alpha : Inport
  F_T : Inport  Port=2
  q : Inport  Port=3
  V : Inport  Port=4
  gamma : Inport  Port=5
  mu : Inport  Port=6
  qbar : Inport  Port=7
  delta_e : Inport  Port=8
  delta_f : Inport  Port=9
  CY : Inport  Port=10
  CL : Subsystem
  Product{,2..4} (4 alike) : Product  RndMeth=Zero
  Product1 : Product  Inputs=3  RndMeth=Zero
  S : Gain  Gain=S
  Sum : Sum  Inputs=|++
  Sum1 : Sum  Inputs=|++
  cos(mu) : Trigonometry  Operator=cos
  sin : Trigonometry
  mV*df_mu(x) : Outport
  wires:
  qbar/1 -> S/1
  S/1 -> Product/1
  Product/1 -> Sum/1  "q_bar*S*(CD*cos(mu)+CL*sin(mu))"
  mu/1 -> sin/1, cos(mu)/1
  Product1/1 -> Sum/2  "F_T*sin(mu)*alpha"
  gamma/1 -> Product2/1
  Sum/1 -> Product2/2
  Product2/1 -> mV*df_mu(x)/1
  F_T/1 -> Product1/3
  sin/1 -> Product1/2, Product4/2  "sin(mu)"
  alpha/1 -> Product1/1, CL/5(alpha)
  delta_f/1 -> CL/2(delta_f)
  delta_e/1 -> CL/1(delta_e)
  Product3/1 -> Sum1/2  "CY*cos(mu)"
  cos(mu)/1 -> Product3/2
  Sum1/1 -> Product/2  "(CY*cos(mu)+CL*sin(mu))"
  q/1 -> CL/3(q)
  V/1 -> CL/4(V)
  CL/1(CL) -> Product4/1
  Product4/1 -> Sum1/1
  CY/1 -> Product3/1

== system cesna_a_37/alpha_beta_mu_controller/sat ==
  mu_set : Inport
  alpha_set : Inport  Port=2
  beta_set : Inport  Port=3
  Mux1 : Mux  Inputs=3
  Saturation1 : Saturate  UpperLimit=pi/4  LowerLimit=-pi/4
  Saturation2 : Saturate  UpperLimit=pi/4  LowerLimit=-pi/4
  Saturation3 : Saturate  UpperLimit=pi/20  LowerLimit=-pi/20
  x_2 : Outport
  wires:
  Mux1/1 -> x_2/1
  mu_set/1 -> Saturation1/1
  alpha_set/1 -> Saturation2/1
  beta_set/1 -> Saturation3/1
  Saturation1/1 -> Mux1/1
  Saturation2/1 -> Mux1/2
  Saturation3/1 -> Mux1/3

== system cesna_a_37/gamma_chi_controller/Calc_CL ==
  alpha : Inport
  delta : Inport  Port=2
  omega : Inport  Port=3
  V : Inport  Port=4
  Add : Sum  Inputs=++++
  CLa : Gain  Gain=CLa
  CLo : Constant  Value=CLo
  Divide : Product  Inputs=*/
  Dot Product : DotProduct  InputSameDT=on  OutDataTypeStr=Inherit: Inherit via internal rule
  "[CLde,CLin]" : Constant  Value=[CLde,CLin]
  "[q]" : Selector  InputPortWidth=3  IndexOptions=Index vector (dialog)  Indices=[2]  OutputSizes=1
  delta_e,f : Selector  InputPortWidth=4  IndexOptions=Index vector (dialog)  Indices=[1,2]  OutputSizes=1
  q*CLq*cbar/2 : Gain  Gain=CLq*cbar/2
  CL : Outport
  wires:
  Add/1 -> CL/1
  Divide/1 -> Add/4
  Dot Product/1 -> Add/3
  CLa/1 -> Add/2
  CLo/1 -> Add/1
  V/1 -> Divide/2
  q*CLq*cbar/2/1 -> Divide/1
  alpha/1 -> CLa/1
  "[q]"/1 -> q*CLq*cbar/2/1
  "[CLde,CLin]"/1 -> Dot Product/1
  delta_e,f/1 -> Dot Product/2
  delta/1 -> delta_e,f/1
  omega/1 -> "[q]"/1

== system cesna_a_37/gamma_chi_controller/Calc_CY ==
  beta : Inport
  delta : Inport  Port=2
  omega : Inport  Port=3
  V : Inport  Port=4
  Add : Sum  Inputs=++++
  CYb : Gain  Gain=CYb
  CYo : Constant  Value=CYo
  Divide : Product  Inputs=*/
  Dot Product : DotProduct  InputSameDT=on  OutDataTypeStr=Inherit: Inherit via internal rule
  Dot Product1 : DotProduct  InputSameDT=on  OutDataTypeStr=Inherit: Inherit via internal rule
  "[CYda,CYdr]" : Constant  Value=[CYda,CYdr]
  "[CYp,CYr]" : Constant  Value=[CYp,CYr]
  "[p,r]" : Selector  InputPortWidth=3  IndexOptions=Index vector (dialog)  Indices=[1,3]  OutputSizes=1
  b/2 : Gain  Gain=b/2
  delta_a,r : Selector  InputPortWidth=4  IndexOptions=Index vector (dialog)  Indices=[3,4]  OutputSizes=1
  CY : Outport
  wires:
  omega/1 -> "[p,r]"/1
  delta/1 -> delta_a,r/1
  delta_a,r/1 -> Dot Product/2
  "[CYda,CYdr]"/1 -> Dot Product/1
  "[CYp,CYr]"/1 -> Dot Product1/1
  "[p,r]"/1 -> Dot Product1/2
  beta/1 -> CYb/1
  Dot Product1/1 -> b/2/1
  b/2/1 -> Divide/1
  V/1 -> Divide/2
  CYo/1 -> Add/1
  CYb/1 -> Add/2
  Dot Product/1 -> Add/3
  Divide/1 -> Add/4
  Add/1 -> CY/1

== system cesna_a_37/gamma_chi_controller/Hz_ipesh ==
  u : Inport
  Discrete State-Space : DiscreteStateSpace  A=A  B=B  C=C  D=D  X0=x0  SampleTime=Ts
  y : Outport
  wires:
  u/1 -> Discrete State-Space/1
  Discrete State-Space/1 -> y/1

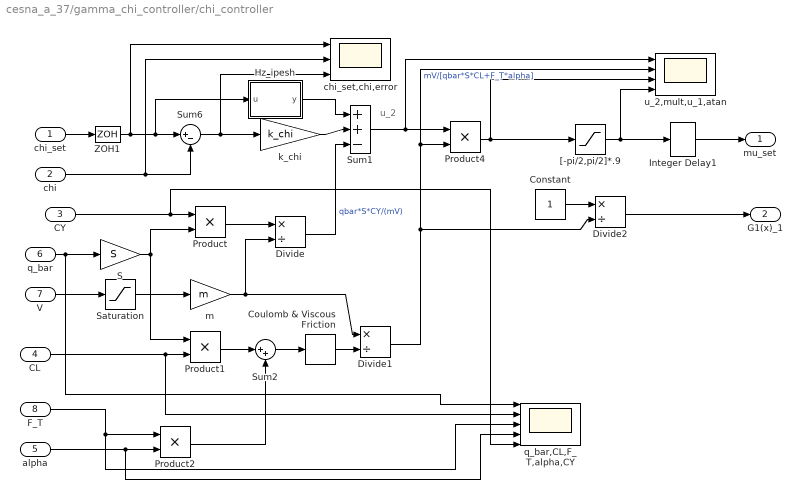
== system cesna_a_37/gamma_chi_controller/chi_controller ==
  note: u_2
  chi_set : Inport
  chi : Inport  Port=2
  CY : Inport  Port=3
  CL : Inport  Port=4
  alpha : Inport  Port=5
  q_bar : Inport  Port=6
  V : Inport  Port=7
  F_T : Inport  Port=8
  Constant : Constant
  Coulomb & Viscous Friction : simulink/Discontinuities/Coulomb & Viscous Friction  SystemSampleTime=-1  offset=.01  gain=1
  Divide : Product  Inputs=*/
  Divide1 : Product  Inputs=*/
  Divide2 : Product  Inputs=*/
  Hz_ipesh : Subsystem  mask{num=[1,0], den=[10*Ts/pi,1], Ts=Ts, y0=0}
      mask prompts: num "Hs num [num]"; den "Hs den [den]"; Ts "Sample Period (s) [Ts]"; y0 "y0 (N)"
      mask init:
      | Hs=tf(num,den);
      | Hz=ipesh_transform(Hs,Ts);
      | [A,B,C,D]=tf2ss(Hz.num{1},Hz.den{1});
      | x0=y0/C;
  Integer Delay1 : simulink/Discrete/Integer Delay  vinit=0.0  samptime=-1  NumDelays=1
  Product{,1..2,4} (4 alike) : Product  RndMeth=Zero
  S : Gain  Gain=S
  Saturation : Saturate  UpperLimit=inf  LowerLimit=10
  Sum1 : Sum  Inputs=|++-
  Sum2 : Sum  Inputs=|++
  Sum6 : Sum  Inputs=|+-
  ZOH1 : ZeroOrderHold  SampleTime=Ts
  "[-pi/2,pi/2]*.9" : Saturate  UpperLimit=.9*pi/2  LowerLimit=-.9*pi/2
  chi_set,chi,error : Scope  NumInputPorts=3
      settings: YMin=0~-0.05~-0.0075  YMax=0.5~0.55~0.02  SaveName=chi_s  SampleInput=on  SampleTime=0.05
  k_chi : Gain  Gain=k_chi
  m : Gain  Gain=m
  q_bar,CL,F_T,alpha,CY : Scope  NumInputPorts=5
      settings: YMin=9000~0.1~0~-0.025~-0.035  YMax=12500~0.23~25000~0.005~0.005  SaveName=ScopeData11  SampleInput=on  SampleTime=0.05
  u_2,mult,u_1,atan : Scope  NumInputPorts=4
      settings: YMin=-0.001~9.7~-0.01~-0.01  YMax=0.003~11~0.03~0.03  SaveName=ScopeData8  SampleInput=on  SampleTime=0.04
  mu_set : Outport
  G1(x)_1 : Outport  Port=2
  wires:
  Sum6/1 -> k_chi/1, chi_set,chi,error/3
  ZOH1/1 -> chi_set,chi,error/1, Sum6/1, Hz_ipesh/1(u)
  chi_set/1 -> ZOH1/1
  chi/1 -> Sum6/2, chi_set,chi,error/2
  CY/1 -> Product/1, q_bar,CL,F_T,alpha,CY/5
  q_bar/1 -> S/1, q_bar,CL,F_T,alpha,CY/1
  V/1 -> Saturation/1
  m/1 -> Divide/2, Divide1/1
  S/1 -> Product/2, Product1/1
  Product/1 -> Divide/1
  alpha/1 -> Product2/2, q_bar,CL,F_T,alpha,CY/4
  Product1/1 -> Sum2/1
  Sum2/1 -> Coulomb & Viscous Friction/1
  Sum1/1 -> Product4/1, u_2,mult,u_1,atan/1
  Divide1/1 -> Product4/2, u_2,mult,u_1,atan/2, Divide2/2  "mV/[qbar*S*CL+F_T*alpha]"
  Product4/1 -> u_2,mult,u_1,atan/3, "[-pi/2,pi/2]*.9"/1
  "[-pi/2,pi/2]*.9"/1 -> Integer Delay1/1, u_2,mult,u_1,atan/4
  Coulomb & Viscous Friction/1 -> Divide1/2
  Saturation/1 -> m/1
  CL/1 -> Product1/2, q_bar,CL,F_T,alpha,CY/2
  F_T/1 -> Product2/1, q_bar,CL,F_T,alpha,CY/3
  Product2/1 -> Sum2/2
  Integer Delay1/1 -> mu_set/1
  k_chi/1 -> Sum1/2
  Divide/1 -> Sum1/3  "qbar*S*CY/(mV)"
  Hz_ipesh/1(y) -> Sum1/1
  Divide2/1 -> G1(x)_1/1
  Constant/1 -> Divide2/1

== system cesna_a_37/gamma_chi_mu_sensor/calc_chi ==
  v_I1 : Inport
  v_I2 : Inport  Port=2
  Divide : Product  Inputs=*/
  Dot Product : DotProduct  InputSameDT=on  OutDataTypeStr=Inherit: Inherit via internal rule
  Math Function : Math  Operator=sqrt  SaturateOnIntegerOverflow=on
  Mux : Mux  Inputs=2
  asin : Trigonometry  Operator=asin
  chi : Outport
  wires:
  v_I1/1 -> Mux/1
  v_I2/1 -> Mux/2, Divide/1
  Mux/1 -> Dot Product/1, Dot Product/2
  Dot Product/1 -> Math Function/1
  Math Function/1 -> Divide/2
  Divide/1 -> asin/1
  asin/1 -> chi/1

== system cesna_a_37/gamma_chi_mu_sensor/calc_gamma ==
  v_I3 : Inport
  V : Inport  Port=2
  Divide : Product  Inputs=*/
  Gain : Gain  Gain=-1
  Trigonometric Function : Trigonometry  Operator=asin
  gamma : Outport
  wires:
  Divide/1 -> Gain/1
  Gain/1 -> Trigonometric Function/1
  v_I3/1 -> Divide/1
  Trigonometric Function/1 -> gamma/1
  V/1 -> Divide/2

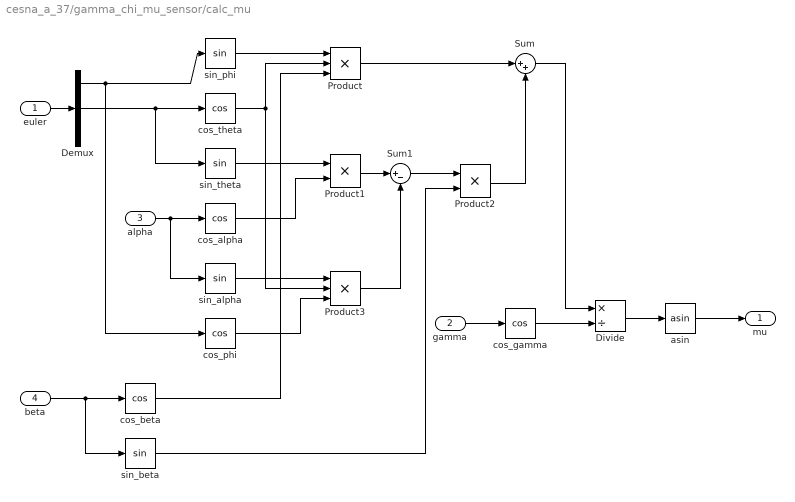
== system cesna_a_37/gamma_chi_mu_sensor/calc_mu ==
  euler : Inport
  gamma : Inport  Port=2
  alpha : Inport  Port=3
  beta : Inport  Port=4
  Demux : Demux  Outputs=3
  Divide : Product  Inputs=*/
  Product : Product  Inputs=3  RndMeth=Zero
  Product1 : Product  RndMeth=Zero
  Product2 : Product  RndMeth=Zero
  Product3 : Product  Inputs=3  RndMeth=Zero
  Sum : Sum  Inputs=|++
  Sum1 : Sum  Inputs=|+-
  asin : Trigonometry  Operator=asin
  cos_alpha : Trigonometry  Operator=cos
  cos_beta : Trigonometry  Operator=cos
  cos_gamma : Trigonometry  Operator=cos
  cos_phi : Trigonometry  Operator=cos
  cos_theta : Trigonometry  Operator=cos
  sin_alpha : Trigonometry
  sin_beta : Trigonometry
  sin_phi : Trigonometry
  sin_theta : Trigonometry
  mu : Outport
  wires:
  gamma/1 -> cos_gamma/1
  cos_gamma/1 -> Divide/2
  Divide/1 -> asin/1
  euler/1 -> Demux/1
  alpha/1 -> cos_alpha/1, sin_alpha/1
  Demux/2 -> cos_theta/1, sin_theta/1
  Demux/1 -> sin_phi/1, cos_phi/1
  sin_phi/1 -> Product/1
  cos_theta/1 -> Product/2, Product3/2
  sin_theta/1 -> Product1/1
  Product/1 -> Sum/1
  Sum/1 -> Divide/1
  beta/1 -> cos_beta/1, sin_beta/1
  cos_beta/1 -> Product/3
  cos_alpha/1 -> Product1/2
  asin/1 -> mu/1
  Product1/1 -> Sum1/1
  Sum1/1 -> Product2/1
  sin_beta/1 -> Product2/2
  sin_alpha/1 -> Product3/1
  cos_phi/1 -> Product3/3
  Product3/1 -> Sum1/2
  Product2/1 -> Sum/2

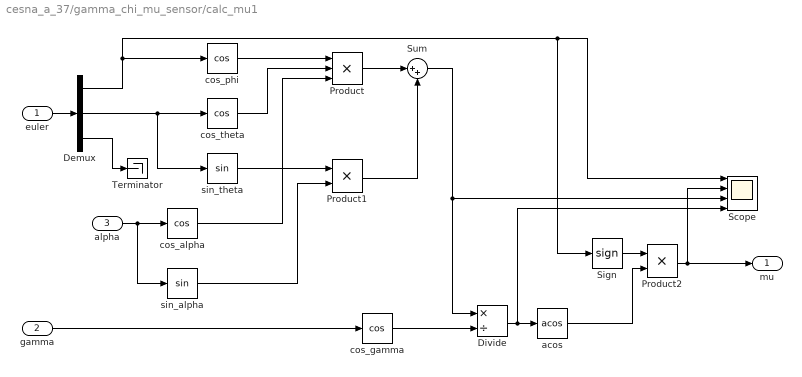
== system cesna_a_37/gamma_chi_mu_sensor/calc_mu1 ==
  euler : Inport
  gamma : Inport  Port=2
  alpha : Inport  Port=3
  Demux : Demux  Outputs=3
  Divide : Product  Inputs=*/
  Product : Product  Inputs=3  RndMeth=Zero
  Product1 : Product  RndMeth=Zero
  Product2 : Product  RndMeth=Zero
  Scope : Scope  NumInputPorts=4
      settings: YMin=-5~-5~-5~-5  YMax=5~5~5~5  SaveName=ScopeData6  SampleInput=on  SampleTime=.01
  Sign : Signum
  Sum : Sum  Inputs=|++
  Terminator : Terminator
  acos : Trigonometry  Operator=acos
  cos_alpha : Trigonometry  Operator=cos
  cos_gamma : Trigonometry  Operator=cos
  cos_phi : Trigonometry  Operator=cos
  cos_theta : Trigonometry  Operator=cos
  sin_alpha : Trigonometry
  sin_theta : Trigonometry
  mu : Outport
  wires:
  Product2/1 -> Scope/2, mu/1
  acos/1 -> Product2/2
  Sign/1 -> Product2/1
  Sum/1 -> Scope/3, Divide/1
  Product1/1 -> Sum/2
  Product/1 -> Sum/1
  sin_alpha/1 -> Product1/2
  sin_theta/1 -> Product1/1
  cos_alpha/1 -> Product/3
  cos_theta/1 -> Product/2
  cos_phi/1 -> Product/1
  Demux/3 -> Terminator/1
  Demux/1 -> Sign/1, Scope/1, cos_phi/1
  Demux/2 -> sin_theta/1, cos_theta/1
  alpha/1 -> sin_alpha/1, cos_alpha/1
  euler/1 -> Demux/1
  Divide/1 -> Scope/4, acos/1
  cos_gamma/1 -> Divide/2
  gamma/1 -> cos_gamma/1

== system cesna_a_37/gamma_chi_mu_sensor/gravity model ==
  h : Inport
  Divide : Product  Inputs=*/
  Dot Product1 : DotProduct  InputSameDT=on  OutDataTypeStr=Inherit: Inherit via internal rule
  Model Info : simulink/Model-Wide Utilities/Model Info  SystemSampleTime=-1  InitialBlockCM=None  BlockCM=None  Frame=on  DisplayStringWithTags=g = g_o [R/(R+h)]^2  HorizontalTextAlignment=Center  LeftAlignmentValue=0.5  SourceBlockDiagram=cesna_a_37  TagMaxNumber=20
  R = Radius of Earth (m) : Constant  Value=6356e3  SampleTime=Ts
  Sum : Sum  Inputs=|++
  g_o : Gain  Gain=9.80665
  g : Outport
  wires:
  g_o/1 -> g/1
  h/1 -> Sum/1
  Dot Product1/1 -> g_o/1
  Divide/1 -> Dot Product1/2, Dot Product1/1
  Sum/1 -> Divide/2
  R = Radius of Earth (m)/1 -> Divide/1, Sum/2

== system cesna_a_37/omega_controller/alg_loop_filt ==
  u : Inport
  Demux : Demux  Outputs=3
  Hz_ipesh : Subsystem  mask{num=[1], den=[10*Ts/pi,1], Ts=Ts, y0=0}
      mask prompts: num "Hs num [num]"; den "Hs den [den]"; Ts "Sample Period (s) [Ts]"; y0 "y0 (N)"
      mask init:
      | Hs=tf(num,den);
      | Hz=ipesh_transform(Hs,Ts);
      | [A,B,C,D]=tf2ss(Hz.num{1},Hz.den{1});
      | x0=y0/C;
  Hz_ipesh1 : Subsystem  mask{num=[1,0], den=[10*Ts/pi,1], Ts=Ts, y0=0}
      mask prompts: num "Hs num [num]"; den "Hs den [den]"; Ts "Sample Period (s) [Ts]"; y0 "y0 (N)"
      mask init:
      | Hs=tf(num,den);
      | Hz=ipesh_transform(Hs,Ts);
      | [A,B,C,D]=tf2ss(Hz.num{1},Hz.den{1});
      | x0=y0/C;
  Hz_ipesh2 : Subsystem  mask{num=[1,0], den=[10*Ts/pi,1], Ts=Ts, y0=0}
      mask prompts: num "Hs num [num]"; den "Hs den [den]"; Ts "Sample Period (s) [Ts]"; y0 "y0 (N)"
      mask init:
      | Hs=tf(num,den);
      | Hz=ipesh_transform(Hs,Ts);
      | [A,B,C,D]=tf2ss(Hz.num{1},Hz.den{1});
      | x0=y0/C;
  Mux2 : Mux  Inputs=3
  y : Outport
  wires:
  u/1 -> Demux/1
  Demux/1 -> Hz_ipesh/1(u)
  Hz_ipesh/1(y) -> Mux2/1
  Demux/2 -> Hz_ipesh1/1(u)
  Hz_ipesh1/1(y) -> Mux2/2
  Demux/3 -> Hz_ipesh2/1(u)
  Hz_ipesh2/1(y) -> Mux2/3
  Mux2/1 -> y/1

== system cesna_a_37/omega_controller/omega_set_dot ==
  omega_set : Inport
  Demux : Demux  Outputs=3
  Hz_ipesh : Subsystem  mask{num=[1,0], den=[10*Ts/pi,1], Ts=Ts, y0=0}
      mask prompts: num "Hs num [num]"; den "Hs den [den]"; Ts "Sample Period (s) [Ts]"; y0 "y0 (N)"
      mask init:
      | Hs=tf(num,den);
      | Hz=ipesh_transform(Hs,Ts);
      | [A,B,C,D]=tf2ss(Hz.num{1},Hz.den{1});
      | x0=y0/C;
  Hz_ipesh1 : Subsystem  mask{num=[1,0], den=[10*Ts/pi,1], Ts=Ts, y0=0}
      mask prompts: num "Hs num [num]"; den "Hs den [den]"; Ts "Sample Period (s) [Ts]"; y0 "y0 (N)"
      mask init:
      | Hs=tf(num,den);
      | Hz=ipesh_transform(Hs,Ts);
      | [A,B,C,D]=tf2ss(Hz.num{1},Hz.den{1});
      | x0=y0/C;
  Hz_ipesh2 : Subsystem  mask{num=[1,0], den=[10*Ts/pi,1], Ts=Ts, y0=0}
      mask prompts: num "Hs num [num]"; den "Hs den [den]"; Ts "Sample Period (s) [Ts]"; y0 "y0 (N)"
      mask init:
      | Hs=tf(num,den);
      | Hz=ipesh_transform(Hs,Ts);
      | [A,B,C,D]=tf2ss(Hz.num{1},Hz.den{1});
      | x0=y0/C;
  Mux2 : Mux  Inputs=3
  omega_set_dot : Outport
  wires:
  omega_set/1 -> Demux/1
  Demux/1 -> Hz_ipesh/1(u)
  Hz_ipesh/1(y) -> Mux2/1
  Demux/2 -> Hz_ipesh1/1(u)
  Hz_ipesh1/1(y) -> Mux2/2
  Demux/3 -> Hz_ipesh2/1(u)
  Hz_ipesh2/1(y) -> Mux2/3
  Mux2/1 -> omega_set_dot/1

== system cesna_a_37/veocity_controller/Dynamic Pressure ==
  V : Inport
  Air Density : Inport  Port=2
  1/2rhoV^2 : Gain  Gain=1/2  SaturateOnIntegerOverflow=on  OutDataTypeStr=Inherit: Same as input  ParamDataTypeStr=Inherit: Same as input
  Product1 : Product  SaturateOnIntegerOverflow=on  InputSameDT=on  OutDataTypeStr=Inherit: Same as first input
  Product2 : Product  SaturateOnIntegerOverflow=on  InputSameDT=on  OutDataTypeStr=Inherit: Same as first input
  qbar : Outport  InitialOutput=0
  wires:
  1/2rhoV^2/1 -> qbar/1
  Product2/1 -> 1/2rhoV^2/1
  Air Density/1 -> Product2/2
  Product1/1 -> Product2/1
  V/1 -> Product1/1, Product1/2

== system cesna_a_37/veocity_controller/Hz_ipesh ==
  u : Inport
  Discrete State-Space : DiscreteStateSpace  A=A  B=B  C=C  D=D  X0=x0  SampleTime=Ts
  y : Outport
  wires:
  u/1 -> Discrete State-Space/1
  Discrete State-Space/1 -> y/1

== system cesna_a_37/veocity_controller/Vs_filt ==
  u : Inport
  Discrete State-Space : DiscreteStateSpace  A=A  B=B  C=C  D=D  X0=x0  SampleTime=Ts
  y : Outport
  wires:
  Discrete State-Space/1 -> y/1
  u/1 -> Discrete State-Space/1

== system cesna_a_37/veocity_controller/anti_windup_control ==
  In1 : Inport
  Add4 : Sum  Inputs=+-
  Hz_ideal_plant : Subsystem  mask{num=[1], den=m*[1,omega_d], Ts=Ts, y0=0}
      mask prompts: num "Hs num [num]"; den "Hs den [den]"; Ts "Sample Period (s) [Ts]"; y0 "y0 (N)"
      mask init:
      | Hs=tf(num,den);
      | Hz=ipesh_transform(Hs,Ts);
      | [A,B,C,D]=tf2ss(Hz.num{1},Hz.den{1});
      | x0=y0/C;
  Saturation : Saturate  UpperLimit=inf  LowerLimit=0
  Out1 : Outport
  Out2 : Outport  Port=2
  wires:
  In1/1 -> Add4/1, Saturation/1
  Saturation/1 -> Add4/2, Out1/1
  Add4/1 -> Hz_ideal_plant/1(u)
  Hz_ideal_plant/1(y) -> Out2/1

== system cesna_a_37/alpha_beta_mu_controller/alg_loop_filt/Hz_ipesh ==
  u : Inport
  Discrete State-Space : DiscreteStateSpace  A=A  B=B  C=C  D=D  X0=x0  SampleTime=Ts
  y : Outport
  wires:
  u/1 -> Discrete State-Space/1
  Discrete State-Space/1 -> y/1

== system cesna_a_37/alpha_beta_mu_controller/alg_loop_filt/Hz_ipesh1 ==
  u : Inport
  Discrete State-Space : DiscreteStateSpace  A=A  B=B  C=C  D=D  X0=x0  SampleTime=Ts
  y : Outport
  wires:
  Discrete State-Space/1 -> y/1
  u/1 -> Discrete State-Space/1

== system cesna_a_37/alpha_beta_mu_controller/alg_loop_filt/Hz_ipesh2 ==
  u : Inport
  Discrete State-Space : DiscreteStateSpace  A=A  B=B  C=C  D=D  X0=x0  SampleTime=Ts
  y : Outport
  wires:
  u/1 -> Discrete State-Space/1
  Discrete State-Space/1 -> y/1

== system cesna_a_37/alpha_beta_mu_controller/mV*delta_f_mu(x)/CL ==
  delta_e : Inport
  delta_f : Inport  Port=2
  q : Inport  Port=3
  V : Inport  Port=4
  alpha : Inport  Port=5
  Add : Sum  Inputs=+++++
  CDo : Constant  Value=CLo
  CLa*alpha : Gain  Gain=CLa
  CLde*delta_e : Gain  Gain=CLde
  CLin*delta_f : Gain  Gain=CLin
  Divide : Product  Inputs=*/
  q*cbar*CLq/2 : Gain  Gain=cbar*CLq/2
  CL : Outport
  wires:
  Divide/1 -> Add/5
  V/1 -> Divide/2
  q*cbar*CLq/2/1 -> Divide/1
  q/1 -> q*cbar*CLq/2/1
  CLa*alpha/1 -> Add/4
  CLin*delta_f/1 -> Add/3
  delta_f/1 -> CLin*delta_f/1
  Add/1 -> CL/1
  alpha/1 -> CLa*alpha/1
  delta_e/1 -> CLde*delta_e/1
  CLde*delta_e/1 -> Add/2
  CDo/1 -> Add/1
